simulink model "DC_DC"  (R2020a)
settings: Solver=VariableStepAuto  StartTime=0.0  StopTime=1  RelTol=1e-3
undefined symbols (not defined in the file): Ion, Lithium
libraries: powerlib x22, androidcommunicationlib x2, electricdrivelib x1, powerlib_meascontrol x1
settings Model: Creator=Kushal Goswami  LastModifiedBy=kushalgoswami
settings DataIOCC: SaveOutput=off  SignalLogging=off  DSMLogging=off  SaveTime=off  ReturnWorkspaceOutputs=off

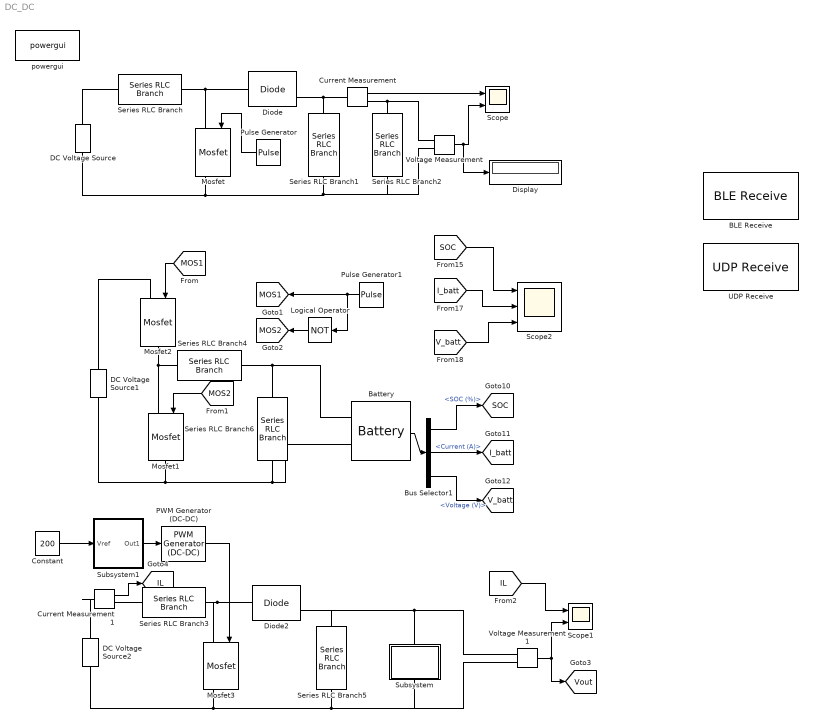
== system DC_DC ==
  BLE Receive : androidcommunicationlib/BLE Receive  DeviceMode=Central (Client)  BluetoothAddress=""  CharUUID=""  ServiceUUID=""  device=No devices  character=No Characteristics  CustomService=off  ServiceName=Heart Rate  CharacteristicName="Heart Rate  Measurement"  CustomServiceUUID=<Enter Service UUID>  CustomCharUUID=<Enter Characteristic UUID>  DataSize=2  SampleTime=0.1  charseruuid=<empty>  seruuid=00001810-0000-1000-8000-00805f9b34fb  PeripheralService=0000180d-0000-1000-8000-00805f9b34fb  PeripheralCharacteristic=00002a37-0000-1000-8000-00805f9b34fb  chruuid=00002a37-0000-1000-8000-00805f9b34fb  Devicename=""  IsCustomService=0
      settings: SourceProductBaseCode=ANDROID
  Battery : electricdrivelib/Extra Sources/Battery  BatType=Lithium-Ion  ShowTempParam=off  ThermalPreset=no  ShowAgeParam=off  NomV=24  NomQ=10  SOC=50  Batt_Tr=1e-4  PresetModel=on  MaxQ=10  MinV=18  FullV=27.9357  Dis_rate=4.3478  R=0.024  Normal_OP=9.0435  expZone="[25.9293     0.491304]"  current=[6.5 13 32.5]  Units=Time  Tci=20  NomT=20  T2=-30  MaxQ2=4.8  FullV2=7.1  Normal_OP2=5.655  expZone2="[6.58           1]"  Rca=0.6  ti=2000  Dp=0  Neq0=0  Tsim=1e6  Ta1=25  Qeol=5.4*0.9  Reol=0.013333*1.2  Char_age=[2.3478, 3]  Dis_age=[2.3478, 10]  N1=1500  N2=10500  N3=1000  N4=1400  Ta2=45  N5=950
  Bus Selector1 : BusSelector  OutputSignals=SOC (%),Current (A),Voltage (V)
  Constant : Constant  Value=200
  Current Measurement : powerlib/Measurements/Current Measurement  PhasorSimulation=off  OutputType=Complex  PSBequivalent=0
  Current Measurement1 : powerlib/Measurements/Current Measurement  PhasorSimulation=off  OutputType=Complex  PSBequivalent=0
  DC Voltage Source : powerlib/Electrical Sources/DC Voltage Source  Amplitude=48  Measurements=None
  DC Voltage Source1 : powerlib/Electrical Sources/DC Voltage Source  Amplitude=48  Measurements=None
  DC Voltage Source2 : powerlib/Electrical Sources/DC Voltage Source  Amplitude=48  Measurements=None
  Diode : powerlib/Power Electronics/Diode  Ron=0.001  Lon=0  Vf=0.8  IC=0  UseSnubber=0  Rs=500  Cs=250e-9  Measurements=on
  Diode2 : powerlib/Power Electronics/Diode  Ron=0.001  Lon=0  Vf=0.8  IC=0  UseSnubber=0  Rs=500  Cs=250e-9  Measurements=on
  Display : Display
  Logical Operator : Logic  Operator=NOT  IconShape=distinctive  AllPortsSameDT=off  OutDataTypeStr=boolean
  Mosfet : powerlib/Power Electronics/Mosfet  Ron=0.1  Lon=0  Rd=0.01  Vfd=0  IC=0  Rs=1e5  Cs=inf  Measurements=on
  Mosfet1 : powerlib/Power Electronics/Mosfet  Ron=0.1  Lon=0  Rd=0.01  Vfd=0  IC=0  Rs=1e5  Cs=inf  Measurements=off
  Mosfet2 : powerlib/Power Electronics/Mosfet  Ron=0.1  Lon=0  Rd=0.01  Vfd=0  IC=0  Rs=1e5  Cs=inf  Measurements=off
  Mosfet3 : powerlib/Power Electronics/Mosfet  Ron=0.1  Lon=0  Rd=0.01  Vfd=0  IC=0  Rs=1e5  Cs=inf  Measurements=on
  PWM Generator (DC-DC) : powerlib_meascontrol/Pulse & Signal Generators/PWM Generator (DC-DC)  Fsw=5000  Ts=0
  Pulse Generator : DiscretePulseGenerator  PulseType=Time based  Period=2.5e-5  PulseWidth=20
  Pulse Generator1 : DiscretePulseGenerator  PulseType=Time based  Period=1e-4  PulseWidth=60
  Scope : Scope  NumInputPorts=2
  Scope1 : Scope  NumInputPorts=2
  Scope2 : Scope  NumInputPorts=3
  Series RLC Branch : powerlib/Elements/Series RLC Branch  LConnTagsString=__new0  RConnTagsString=__new0  BranchType=L  Resistance=1  Inductance=2e-5  SetiL0=off  InitialCurrent=0  Capacitance=1e-6  Setx0=off  InitialVoltage=0  Measurements=None
  Series RLC Branch1 : powerlib/Elements/Series RLC Branch  LConnTagsString=__new0  RConnTagsString=__new0  BranchType=C  Resistance=1  Inductance=1e-3  SetiL0=off  InitialCurrent=0  Capacitance=1e-5  Setx0=off  InitialVoltage=0  Measurements=None
  Series RLC Branch2 : powerlib/Elements/Series RLC Branch  LConnTagsString=__new0  RConnTagsString=__new0  BranchType=R  Resistance=10  Inductance=1e-3  SetiL0=off  InitialCurrent=0  Capacitance=1e-6  Setx0=off  InitialVoltage=0  Measurements=None
  Series RLC Branch3 : powerlib/Elements/Series RLC Branch  LConnTagsString=__new0  RConnTagsString=__new0  BranchType=L  Resistance=1  Inductance=2e-5  SetiL0=off  InitialCurrent=0  Capacitance=1e-6  Setx0=off  InitialVoltage=0  Measurements=None
  Series RLC Branch4 : powerlib/Elements/Series RLC Branch  LConnTagsString=__new0  RConnTagsString=__new0  BranchType=RL  Resistance=0.05  Inductance=5.76e-2  SetiL0=off  InitialCurrent=0  Capacitance=1e-6  Setx0=off  InitialVoltage=0  Measurements=None
  Series RLC Branch5 : powerlib/Elements/Series RLC Branch  LConnTagsString=__new0  RConnTagsString=__new0  BranchType=C  Resistance=1  Inductance=1e-3  SetiL0=off  InitialCurrent=0  Capacitance=1e-5  Setx0=off  InitialVoltage=0  Measurements=None
  Series RLC Branch6 : powerlib/Elements/Series RLC Branch  LConnTagsString=__new0  RConnTagsString=__new0  BranchType=RC  Resistance=0.001  Inductance=5.76e-4  SetiL0=off  InitialCurrent=0  Capacitance=1000e-6  Setx0=off  InitialVoltage=0  Measurements=None
  Subsystem : Subsystem
  Subsystem1 : Subsystem
  UDP Receive : androidcommunicationlib/UDP Receive  localURL='0.0.0.0'  localPort=25000  remoteURL='0.0.0.0'  remotePort=-1  recvBufferSize=8192  signalDatatype=uint8  dims=255  isVarSize=off  showBlockingTime=off  blockingTime=0  sampletime=0.01  blockPlatform=Android
      settings: SourceProductBaseCode=ANDROID
  Voltage Measurement : powerlib/Measurements/Voltage Measurement  PhasorSimulation=off  OutputType=Complex  PSBequivalent=0
  Voltage Measurement1 : powerlib/Measurements/Voltage Measurement  PhasorSimulation=off  OutputType=Complex  PSBequivalent=0
  powergui : powerlib/powergui  Priority=1  SimulationMode=Discrete  SampleTime=1e-6  frequency=60  Iterations=50  frequencyindice=0  Pbase=100e6  ErrMax=1e-4  UnitsV=kV  UnitsW=MW  buscounter=0  FunctionMessages=off  echomessages=off  EnableUseOfTLC=off  CurrentSourceSwitches=off  DisableSnubberDevices=off  DisableRonSwitches=off  DisableVfSwitches=off  DisplayEquations=off  AutomaticDiscreteSolvers=off  SolverType=Tustin/Backward Euler (TBE)  Interpol=off  ExternalGateDelay=off  methode=off  Ts=100  x0status=blocks  SPID=on  SwTol=0  HookPort=off  NonlinearTolerance=1e-4  nMaxIteration=100  ContinueOnMaxIteration=off  RestoreLinks=warning  ResistiveCurrentMeasurement=off  Frange=[0:2:500]  Ylog=off  Xlog=on  ShowGrid=off  save=off  variable=ZData  structure=0  ZoomFFT=off  StartTime=0.0  cycles=1  DisplayStyle=1  fundamental=60  FreqAxis=off  MaxFrequency=1000  frequencyindicesteady=1  RmsSteady=1  display=off
  tag scope: IL=global, I_batt=global, MOS1=global, MOS2=global, SOC=global, V_batt=global, Vout=global
  wires:
  Current Measurement/1 -> Scope/1
  Voltage Measurement/1 -> Display/1, Scope/2
  Pulse Generator/1 -> Mosfet/1
  Bus Selector1/3 -> [V_batt]  "<Voltage (V)>"
  Battery/1 -> Bus Selector1/1
  [SOC] -> Scope2/1
  [V_batt] -> Scope2/3
  Bus Selector1/2 -> [I_batt]  "<Current (A)>"
  [I_batt] -> Scope2/2
  Bus Selector1/1 -> [SOC]  "<SOC (%)>"
  Pulse Generator1/1 -> Logical Operator/1, [MOS1]
  Logical Operator/1 -> [MOS2]
  [MOS1] -> Mosfet2/1
  [MOS2] -> Mosfet1/1
  Voltage Measurement1/1 -> [Vout], Scope1/2
  PWM Generator (DC-DC)/1 -> Mosfet3/1
  Current Measurement1/1 -> [IL]
  [IL] -> Scope1/1
  Constant/1 -> Subsystem1/1(Vref)
  Subsystem1/1(Out1) -> PWM Generator (DC-DC)/1
  connections:
  Diode/LConn1 -- Mosfet/LConn1 -- Series RLC Branch/RConn1
  Series RLC Branch/LConn1 -- DC Voltage Source/RConn1
  DC Voltage Source/LConn1 -- Voltage Measurement/LConn2 -- Series RLC Branch2/RConn1 -- Series RLC Branch1/RConn1 -- Mosfet/RConn1
  Series RLC Branch2/LConn1 -- Voltage Measurement/LConn1 -- Current Measurement/RConn1
  Diode/RConn1 -- Series RLC Branch1/LConn1 -- Current Measurement/LConn1
  Battery/LConn2 -- Series RLC Branch6/RConn1 -- Mosfet1/RConn1 -- DC Voltage Source1/LConn1
  Series RLC Branch4/RConn1 -- Series RLC Branch6/LConn1 -- Battery/LConn1
  Mosfet2/RConn1 -- Mosfet1/LConn1 -- Series RLC Branch4/LConn1
  Mosfet2/LConn1 -- DC Voltage Source1/RConn1
  DC Voltage Source2/LConn1 -- Subsystem/RConn1 -- Voltage Measurement1/LConn2 -- Series RLC Branch5/RConn1 -- Mosfet3/RConn1
  Subsystem/LConn1 -- Series RLC Branch5/LConn1 -- Diode2/RConn1 -- Voltage Measurement1/LConn1
  Series RLC Branch3/RConn1 -- Mosfet3/LConn1 -- Diode2/LConn1
  Current Measurement1/RConn1 -- Series RLC Branch3/LConn1
  Current Measurement1/LConn1 -- DC Voltage Source2/RConn1

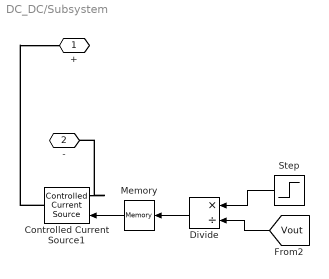
== system DC_DC/Subsystem ==
  Controlled Current Source1 : powerlib/Electrical Sources/Controlled Current Source  Initialize=on  Source_Type=AC  Amplitude=0  Phase=0  Frequency=0  Measurements=None
  Divide : Product  Inputs=*/
  Memory : Memory
  Step : Step  SampleTime=0
  + : PMIOPort  Side=Right
  - : PMIOPort  Port=2  Side=Left
  wires:
  Memory/1 -> Controlled Current Source1/1
  Divide/1 -> Memory/1
  [Vout] -> Divide/2
  Step/1 -> Divide/1
  connections:
  Controlled Current Source1/RConn1 -- +/RConn1
  Controlled Current Source1/LConn1 -- -/RConn1

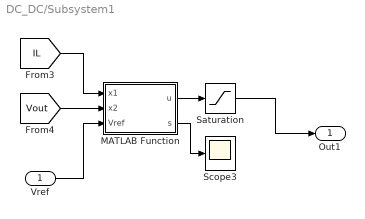
== system DC_DC/Subsystem1 ==
  Vref : Inport
  MATLAB Function : MATLAB Function  TreatAsAtomicUnit=on
  Saturation : Saturate
  Scope3 : Scope
  Out1 : Outport
  wires:
  MATLAB Function/2(s) -> Scope3/1
  MATLAB Function/1(u) -> Saturation/1
  [IL] -> MATLAB Function/1(x1)
  Vref/1 -> MATLAB Function/3(Vref)
  [Vout] -> MATLAB Function/2(x2)
  Saturation/1 -> Out1/1

== matlab function DC_DC/Subsystem1/MATLAB Function ==
  data: x1 input; u output; x2 input; Vref input; s output
function [u,s] = SMC(x1,x2,Vref)
L=1e-3;
C=1000e-6;
P=1000;
E=50;
iref=P/50;
K=50e6;
Lambda=16e4;

s=x1*x2-Vref*iref;
u=1-((P*x1/(C*x2))-E*x2/L-Lambda*s)/(x1^2/C-x2^2/L)+K*sign(s)/(x1^2/C-x2^2/L);
if u<0
    u=0;
end
if u>0.95
    u=0.95;
end
end
